simulink model "test_LLA_FLAT_EARTH"  (R2013b)
settings: Solver=FixedStepDiscrete  StartTime=0.0  StopTime=530  FixedStep=1  RelTol=1e-3
undefined symbols (not defined in the file): Earth, WGS84
libraries: aerolibtransform2 x2, simulink_extras x1
settings Model: Creator=Matteo  LastModifiedBy=Matteo

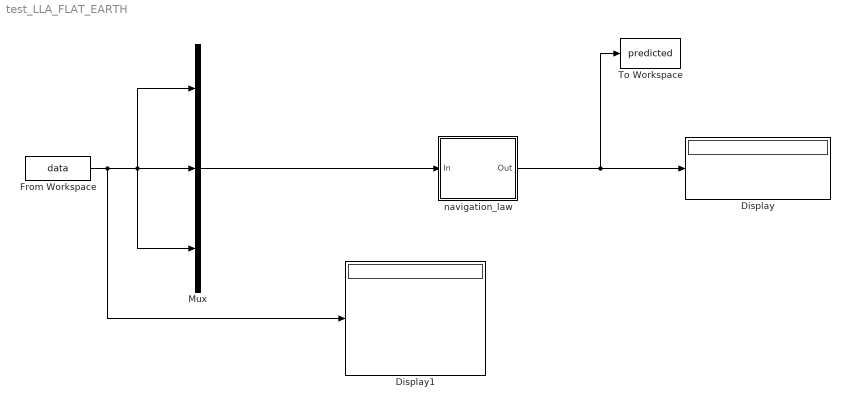
== system test_LLA_FLAT_EARTH ==
  Display : Display
  Display1 : Display
  From Workspace : FromWorkspace  VariableName=data  OutDataTypeStr=double  SampleTime=0
  Mux : Mux  Inputs=[5 5 5 ]
  To Workspace : ToWorkspace  VariableName=predicted  SampleTime=-1
  navigation_law : Subsystem
  wires:
  Mux/1 -> navigation_law/1(In)
  navigation_law/1(Out) -> To Workspace/1, Display/1
  From Workspace/1 -> Display1/1, Mux/3, Mux/1, Mux/2

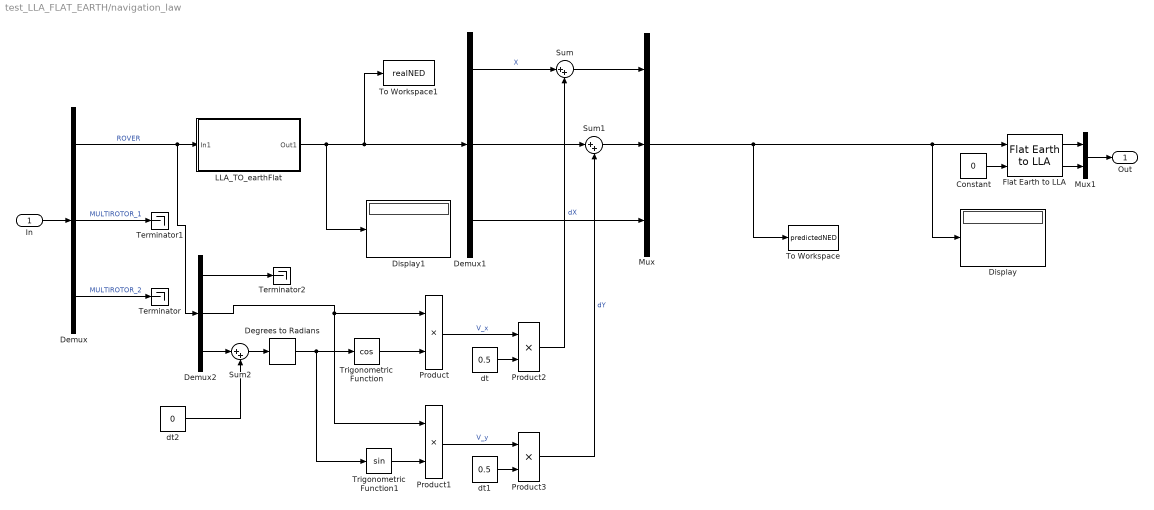
== system test_LLA_FLAT_EARTH/navigation_law ==
  In : Inport
  Constant : Constant  Value=0  OutDataTypeStr=single
  Degrees to Radians : simulink_extras/Transformations/Degrees to Radians
  Demux : Demux  Outputs=[5 5 5]
  Demux1 : Demux  Outputs=3
  Demux2 : Demux  Outputs=[3 1 1]
  Display : Display
  Display1 : Display
  Flat Earth to LLA : aerolibtransform2/Flat Earth to LLA  units=Metric (MKS)  ptype=Earth (WGS84)  F=1/298.257223563  R=6378137  LL0=[44.201892800000003 12.062565800000000]  psi=0
  LLA_TO_earthFlat : Subsystem
  Mux : Mux  Inputs=3
  Mux1 : Mux  Inputs=[2 1]
  Product{,1..3} (4 alike) : Product
  Sum : Sum  Inputs=|++
  Sum1 : Sum  Inputs=|++
  Sum2 : Sum  Inputs=|++
  Terminator : Terminator
  Terminator1 : Terminator
  Terminator2 : Terminator
  To Workspace : ToWorkspace  VariableName=predictedNED  SampleTime=-1
  To Workspace1 : ToWorkspace  VariableName=realNED  SampleTime=-1
  Trigonometric Function : Trigonometry  Operator=cos
  Trigonometric Function1 : Trigonometry
  dt : Constant  Value=0.5
  dt1 : Constant  Value=0.5
  dt2 : Constant  Value=0
  Out : Outport
  wires:
  Mux1/1 -> Out/1
  Flat Earth to LLA/2 -> Mux1/2
  Flat Earth to LLA/1 -> Mux1/1
  Constant/1 -> Flat Earth to LLA/2
  Mux/1 -> To Workspace/1, Display/1, Flat Earth to LLA/1
  Sum1/1 -> Mux/2
  Sum/1 -> Mux/1
  Demux1/3 -> Mux/3
  Demux1/2 -> Sum1/1
  Demux1/1 -> Sum/1  "X"
  Product3/1 -> Sum1/2  "dY"
  dt1/1 -> Product3/2
  Product1/1 -> Product3/1  "V_y"
  Product2/1 -> Sum/2  "dX"
  dt/1 -> Product2/2
  Trigonometric Function1/1 -> Product1/2
  Degrees to Radians/1 -> Trigonometric Function1/1, Trigonometric Function/1
  Product/1 -> Product2/1  "V_x"
  Trigonometric Function/1 -> Product/2
  Demux2/2 -> Product/1, Product1/1
  Demux2/1 -> Terminator2/1
  LLA_TO_earthFlat/1(Out1) -> Display1/1, To Workspace1/1, Demux1/1
  Demux/3 -> Terminator/1  "MULTIROTOR_2"
  In/1 -> Demux/1
  Demux/2 -> Terminator1/1  "MULTIROTOR_1"
  Demux/1 -> Demux2/1, LLA_TO_earthFlat/1(In1)  "ROVER"
  Demux2/3 -> Sum2/1
  Sum2/1 -> Degrees to Radians/1
  dt2/1 -> Sum2/2

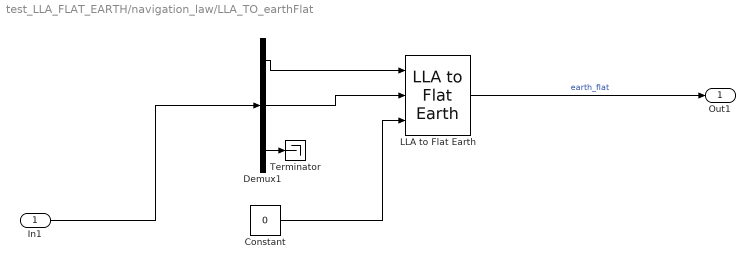
== system test_LLA_FLAT_EARTH/navigation_law/LLA_TO_earthFlat ==
  In1 : Inport
  Constant : Constant  Value=0  OutDataTypeStr=double
  Demux1 : Demux  Outputs=[2 1 2]
  LLA to Flat Earth : aerolibtransform2/LLA to Flat Earth  units=Metric (MKS)  ptype=Earth (WGS84)  F=1/298.257223563  R=6378137  LL0="[44.201892800000003  12.062565800000000]"  psi=0
  Terminator : Terminator
  Out1 : Outport
  wires:
  Constant/1 -> LLA to Flat Earth/3
  Demux1/1 -> LLA to Flat Earth/1
  LLA to Flat Earth/1 -> Out1/1  "earth_flat"
  Demux1/2 -> LLA to Flat Earth/2
  In1/1 -> Demux1/1
  Demux1/3 -> Terminator/1
